simulink model "SWC_HALIN_CDD_type"  (R2021b)
settings: Solver=FixedStepDiscrete  StartTime=0.0  StopTime=10.0  FixedStep=0.005  RelTol=1e-3
undefined symbols (not defined in the file or in its folder): C_TASK_5MS_S, DIDLen_APSFunConfig, DIDLen_AutoLock, DIDLen_AutoWipHSpdEN, DIDLen_DKCKey, DIDLen_DRLDis, DIDLen_DynoMode, DIDLen_FMHTimer, DIDLen_OBDReq, DIDLen_TestGroup, DIDLen_TireSize, DIDLen_TurnLampFLThreCurr, DIDLen_TurnLampFRThreCurr, DIDLen_TurnLampRLThreCurr, DIDLen_TurnLampRRThreCurr, DIDLen_USSConfig, DIDLen_WipRLSCmdCutFilter, DIDLen_WipRLSCmdHoldFilter, DIDLen_XWDMode, DIDNum_APSFunConfig, DIDNum_AutoLock, DIDNum_AutoWipHSpdEN, DIDNum_DKCKey, DIDNum_DRLDis, DIDNum_DynoMode, DIDNum_FMHTimer, DIDNum_OBDReq, DIDNum_TestGroup, DIDNum_TireSize, DIDNum_TurnLampFLThreCurr, DIDNum_TurnLampFRThreCurr, DIDNum_TurnLampRLThreCurr, DIDNum_TurnLampRRThreCurr, DIDNum_USSConfig, DIDNum_WipRLSCmdCutFilter, DIDNum_WipRLSCmdHoldFilter, DIDNum_XWDMode, ENUM_DRIVETRAIN_AWD, ENUM_DRIVETRAIN_FWD, ENUM_DRIVETRAIN_RWD, ENUM_REGENLEVEL_LV1, ENUM_REGENLEVEL_LV2, ENUM_REGENLEVEL_LV3, ENUM_REGENLEVEL_LV4, ENUM_REGENLEVEL_LV5, ENUM_REGENLEVEL_OPD, ENUM_TPMSSTA_FAT, ENUM_TPMSSTA_LOWBATTERY, ENUM_TPMSSTA_TRIGGER, FALSE, FIVE_INT, FOUR_INT, KHAL_CANBusOffDebounce_s, KHAL_DefaultRegenMode_enum, KHAL_DKCDecryptEnable_flg_ovrdflg, KHAL_DKCDecryptEnable_flg_ovrdval, KHAL_RandomNumberY1_enum, KHAL_RandomNumberY2_enum, KHAL_RandomNumberY_ovrdflg, KHAL_TPMSRESBUTT_flg_ovrdflg ... (+9)
libraries: simulink x229, FVT_lib x29, hcu_lib x25, hdlsllib x15
(part 6 of 8)

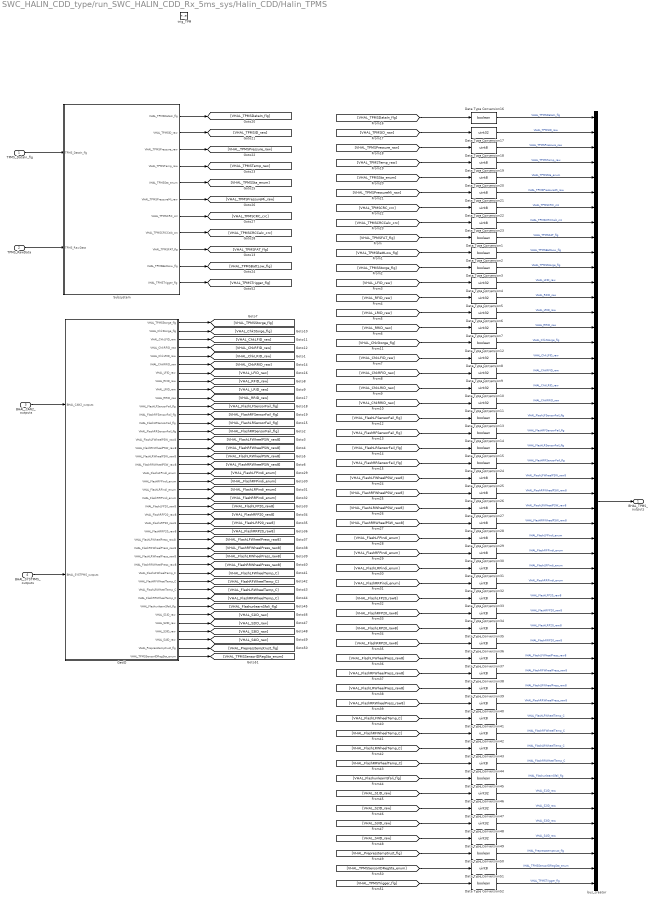
== system SWC_HALIN_CDD_type/run_SWC_HALIN_CDD_Rx_5ms_sys/Halin_CDD/Halin_TPMS ==
  TPMS_DataIn_flg : Inport
  TPMS_RawData : Inport  Port=2
  BHAL_CAN2_outputs : Inport  Port=3
  BHAL_SYSTPMS_outputs : Inport  Port=4
  trig_TPM : TriggerPort  TriggerType=function-call  VariantControl=(inherit)
  Data Type Conversion{1..3,12..16,24,45,50,52} (12 alike) : DataTypeConversion  OutDataTypeStr=boolean
  Data Type Conversion{4..11,17,46..49} (13 alike) : DataTypeConversion  OutDataTypeStr=uint32
  Data Type Conversion{18..23,25..44,51} (27 alike) : DataTypeConversion  OutDataTypeStr=uint8
  GetID : Subsystem
  Subsystem : Subsystem
  bus_creator : BusCreator  Inputs=52  OutDataTypeStr=Bus: BHAL_TPMS_outputs  NonVirtualBus=on
  BHAL_TPMS_outputs : Outport
  wires:
  TPMS_DataIn_flg/1 -> Subsystem/1(TPMS_DataIn_flg)
  Data Type Conversion29/1 -> bus_creator/29  "VHAL_FlashLFPindi_enum"
  GetID/20(VHAL_FlashRFPindi_enum) -> [VHAL_FlashRFPindi_enum]
  GetID/32(VHAL_FlashRFWheelTemp_C) -> [VHAL_FlashRFWheelTemp_C]
  Data Type Conversion2/1 -> bus_creator/10  "VHAL_TPMSBattLow_flg"
  BHAL_CAN2_outputs/1 -> GetID/1(BHAL_CAN2_outputs)
  [VHAL_TPMSBattLow_flg] -> Data Type Conversion2/1
  [VHAL_FlashLRPindi_enum] -> Data Type Conversion31/1
  [VHAL_FlashunlearnSfali_flg] -> Data Type Conversion45/1
  [VHAL_FlashLFPindi_enum] -> Data Type Conversion29/1
  Data Type Conversion28/1 -> bus_creator/28  "VHAL_FlashRRWheelPSW_raw8"
  [VHAL_FlashLFP20_raw8] -> Data Type Conversion33/1
  [VHAL_RRID_raw] -> Data Type Conversion7/1
  Data Type Conversion42/1 -> bus_creator/42  "VHAL_FlashRFWheelTemp_C"
  Data Type Conversion27/1 -> bus_creator/27  "VHAL_FlashLRWheelPSW_raw8"
  [VHAL_FlashLFWheelTemp_C] -> Data Type Conversion41/1
  Data Type Conversion26/1 -> bus_creator/26  "VHAL_FlashRFWheelPSW_raw8"
  [VHAL_FlashRRP20_raw8] -> Data Type Conversion36/1
  GetID/16(VHAL_FlashRFWheelPSW_raw8) -> [VHAL_FlashRFWheelPSW_raw8]
  [VHAL_RFID_raw] -> Data Type Conversion5/1
  Data Type Conversion33/1 -> bus_creator/33  "VHAL_FlashLFP20_raw8"
  Data Type Conversion24/1 -> bus_creator/24  "VHAL_FlashRRSensorFail_flg"
  Data Type Conversion44/1 -> bus_creator/44  "VHAL_FlashRRWheelTemp_C"
  Data Type Conversion34/1 -> bus_creator/34  "VHAL_FlashRFP20_raw8"
  Data Type Conversion45/1 -> bus_creator/45  "VHAL_FlashunlearnSfali_flg"
  GetID/9(VHAL_LRID_raw) -> [VHAL_LRID_raw]
  Data Type Conversion41/1 -> bus_creator/41  "VHAL_FlashLFWheelTemp_C"
  GetID/15(VHAL_FlashLFWheelPSW_raw8) -> [VHAL_FlashLFWheelPSW_raw8]
  Data Type Conversion15/1 -> bus_creator/23  "VHAL_FlashLRSensorFail_flg"
  [VHAL_FlashLRWheelPress_raw8] -> Data Type Conversion39/1
  Data Type Conversion14/1 -> bus_creator/22  "VHAL_FlashRFSensorFail_flg"
  GetID/34(VHAL_FlashRRWheelTemp_C) -> [VHAL_FlashRRWheelTemp_C]
  Data Type Conversion13/1 -> bus_creator/21  "VHAL_FlashLFSensorFail_flg"
  Data Type Conversion32/1 -> bus_creator/32  "VHAL_FlashRRPindi_enum"
  Data Type Conversion31/1 -> bus_creator/31  "VHAL_FlashLRPindi_enum"
  Data Type Conversion16/1 -> bus_creator/1  "VHAL_TPMSDataIn_flg"
  GetID/22(VHAL_FlashRRPindi_enum) -> [VHAL_FlashRRPindi_enum]
  [VHAL_FlashRFSensorFail_flg] -> Data Type Conversion14/1
  GetID/18(VHAL_FlashRRWheelPSW_raw8) -> [VHAL_FlashRRWheelPSW_raw8]
  Data Type Conversion43/1 -> bus_creator/43  "VHAL_FlashLRWheelTemp_C"
  Data Type Conversion22/1 -> bus_creator/7  "VHAL_TPMSCRC_crc"
  Data Type Conversion40/1 -> bus_creator/40  "VHAL_FlashRRWheelPress_raw8"
  Data Type Conversion39/1 -> bus_creator/39  "VHAL_FlashLRWheelPress_raw8"
  [VHAL_FlashRRPindi_enum] -> Data Type Conversion32/1
  Data Type Conversion38/1 -> bus_creator/38  "VHAL_FlashRFWheelPress_raw8"
  [VHAL_FlashLRP20_raw8] -> Data Type Conversion35/1
  Data Type Conversion35/1 -> bus_creator/35  "VHAL_FlashLRP20_raw8"
  GetID/14(VHAL_FlashRRSensorFail_flg) -> [VHAL_FlashRRSensorFail_flg]
  Data Type Conversion37/1 -> bus_creator/37  "VHAL_FlashLFWheelPress_raw8"
  Data Type Conversion36/1 -> bus_creator/36  "VHAL_FlashRRP20_raw8"
  [VHAL_FlashRRWheelTemp_C] -> Data Type Conversion44/1
  [VHAL_FlashLFWheelPress_raw8] -> Data Type Conversion37/1
  GetID/33(VHAL_FlashLRWheelTemp_C) -> [VHAL_FlashLRWheelTemp_C]
  GetID/26(VHAL_FlashRRP20_raw8) -> [VHAL_FlashRRP20_raw8]
  [VHAL_TPMSFAT_flg] -> Data Type Conversion1/1
  [VHAL_TPMSSta_enum] -> Data Type Conversion20/1
  GetID/25(VHAL_FlashLRP20_raw8) -> [VHAL_FlashLRP20_raw8]
  [VHAL_FlashRRWheelPress_raw8] -> Data Type Conversion40/1
  [VHAL_FlashRFP20_raw8] -> Data Type Conversion34/1
  [VHAL_LFID_raw] -> Data Type Conversion4/1
  [VHAL_FlashRFWheelPSW_raw8] -> Data Type Conversion26/1
  [VHAL_FlashRFWheelTemp_C] -> Data Type Conversion42/1
  [VHAL_FlashLRWheelTemp_C] -> Data Type Conversion43/1
  [VHAL_TPMSCRCCalc_crc] -> Data Type Conversion23/1
  GetID/31(VHAL_FlashLFWheelTemp_C) -> [VHAL_FlashLFWheelTemp_C]
  [VHAL_FlashRRSensorFail_flg] -> Data Type Conversion24/1
  [VHAL_FlashLFSensorFail_flg] -> Data Type Conversion13/1
  GetID/30(VHAL_FlashRRWheelPress_raw8) -> [VHAL_FlashRRWheelPress_raw8]
  Data Type Conversion3/1 -> bus_creator/11  "VHAL_TPMSStorge_flg"
  GetID/29(VHAL_FlashLRWheelPress_raw8) -> [VHAL_FlashLRWheelPress_raw8]
  GetID/21(VHAL_FlashLRPindi_enum) -> [VHAL_FlashLRPindi_enum]
  GetID/1(VHAL_TPMSStorge_flg) -> [VHAL_TPMSStorge_flg]
  [VHAL_FlashRFPindi_enum] -> Data Type Conversion30/1
  GetID/19(VHAL_FlashLFPindi_enum) -> [VHAL_FlashLFPindi_enum]
  GetID/23(VHAL_FlashLFP20_raw8) -> [VHAL_FlashLFP20_raw8]
  Data Type Conversion6/1 -> bus_creator/14  "VHAL_LRID_raw"
  GetID/6(VHAL_ChkRRID_raw) -> [VHAL_ChkRRID_raw]
  [VHAL_TPMSDataIn_flg] -> Data Type Conversion16/1
  GetID/17(VHAL_FlashLRWheelPSW_raw8) -> [VHAL_FlashLRWheelPSW_raw8]
  [VHAL_FlashRFWheelPress_raw8] -> Data Type Conversion38/1
  Data Type Conversion1/1 -> bus_creator/9  "VHAL_TPMSFAT_flg"
  GetID/3(VHAL_ChkLFID_raw) -> [VHAL_ChkLFID_raw]
  GetID/35(VHAL_FlashunlearnSfali_flg) -> [VHAL_FlashunlearnSfali_flg]
  [VHAL_FlashLFWheelPSW_raw8] -> Data Type Conversion25/1
  GetID/8(VHAL_RFID_raw) -> [VHAL_RFID_raw]
  GetID/10(VHAL_RRID_raw) -> [VHAL_RRID_raw]
  Data Type Conversion12/1 -> bus_creator/16  "VHAL_ChkStorge_flg"
  [VHAL_FlashLRWheelPSW_raw8] -> Data Type Conversion27/1
  GetID/7(VHAL_LFID_raw) -> [VHAL_LFID_raw]
  Data Type Conversion18/1 -> bus_creator/3  "VHAL_TPMSPressure_raw"
  Data Type Conversion9/1 -> bus_creator/18  "VHAL_ChkRFID_raw"
  Data Type Conversion10/1 -> bus_creator/19  "VHAL_ChkLRID_raw"
  GetID/11(VHAL_FlashLFSensorFail_flg) -> [VHAL_FlashLFSensorFail_flg]
  GetID/27(VHAL_FlashLFWheelPress_raw8) -> [VHAL_FlashLFWheelPress_raw8]
  Data Type Conversion11/1 -> bus_creator/20  "VHAL_ChkRRID_raw"
  Data Type Conversion7/1 -> bus_creator/15  "VHAL_RRID_raw"
  GetID/4(VHAL_ChkRFID_raw) -> [VHAL_ChkRFID_raw]
  [VHAL_TPMSID_raw] -> Data Type Conversion17/1
  [VHAL_ChkStorge_flg] -> Data Type Conversion12/1
  GetID/28(VHAL_FlashRFWheelPress_raw8) -> [VHAL_FlashRFWheelPress_raw8]
  Data Type Conversion8/1 -> bus_creator/17  "VHAL_ChkLFID_raw"
  [VHAL_ChkRRID_raw] -> Data Type Conversion11/1
  Data Type Conversion4/1 -> bus_creator/12  "VHAL_LFID_raw"
  [VHAL_ChkLRID_raw] -> Data Type Conversion10/1
  [VHAL_ChkLFID_raw] -> Data Type Conversion8/1
  [VHAL_ChkRFID_raw] -> Data Type Conversion9/1
  Data Type Conversion5/1 -> bus_creator/13  "VHAL_RFID_raw"
  [VHAL_LRID_raw] -> Data Type Conversion6/1
  [VHAL_TPMSStorge_flg] -> Data Type Conversion3/1
  GetID/2(VHAL_ChkStorge_flg) -> [VHAL_ChkStorge_flg]
  [VHAL_TPMSCRC_crc] -> Data Type Conversion22/1
  Data Type Conversion19/1 -> bus_creator/4  "VHAL_TPMSTemp_raw"
  BHAL_SYSTPMS_outputs/1 -> GetID/2(BHAL_SYSTPMS_outputs)
  [VHAL_FlashLRSensorFail_flg] -> Data Type Conversion15/1
  Data Type Conversion17/1 -> bus_creator/2  "VHAL_TPMSID_raw"
  Data Type Conversion23/1 -> bus_creator/8  "VHAL_TPMSCRCCalc_crc"
  Data Type Conversion30/1 -> bus_creator/30  "VHAL_FlashRFPindi_enum"
  Data Type Conversion21/1 -> bus_creator/6  "VHAL_TPMSPressureMi_raw"
  GetID/5(VHAL_ChkLRID_raw) -> [VHAL_ChkLRID_raw]
  [VHAL_TPMSTemp_raw] -> Data Type Conversion19/1
  GetID/13(VHAL_FlashLRSensorFail_flg) -> [VHAL_FlashLRSensorFail_flg]
  [VHAL_TPMSPressure_raw] -> Data Type Conversion18/1
  GetID/24(VHAL_FlashRFP20_raw8) -> [VHAL_FlashRFP20_raw8]
  bus_creator/1 -> BHAL_TPMS_outputs/1
  Data Type Conversion20/1 -> bus_creator/5  "VHAL_TPMSSta_enum"
  Data Type Conversion25/1 -> bus_creator/25  "VHAL_FlashLFWheelPSW_raw8"
  [VHAL_TPMSPressureMi_raw] -> Data Type Conversion21/1
  GetID/12(VHAL_FlashRFSensorFail_flg) -> [VHAL_FlashRFSensorFail_flg]
  [VHAL_FlashRRWheelPSW_raw8] -> Data Type Conversion28/1
  GetID/36(VHAL_S1ID_raw) -> [VHAL_S1ID_raw]
  GetID/37(VHAL_S2ID_raw) -> [VHAL_S2ID_raw]
  GetID/38(VHAL_S3ID_raw) -> [VHAL_S3ID_raw]
  GetID/39(VHAL_S4ID_raw) -> [VHAL_S4ID_raw]
  Data Type Conversion46/1 -> bus_creator/46  "VHAL_S1ID_raw"
  Data Type Conversion49/1 -> bus_creator/49  "VHAL_S4ID_raw"
  Data Type Conversion48/1 -> bus_creator/48  "VHAL_S3ID_raw"
  Data Type Conversion47/1 -> bus_creator/47  "VHAL_S2ID_raw"
  [VHAL_S1ID_raw] -> Data Type Conversion46/1
  [VHAL_S2ID_raw] -> Data Type Conversion47/1
  [VHAL_S3ID_raw] -> Data Type Conversion48/1
  [VHAL_S4ID_raw] -> Data Type Conversion49/1
  GetID/40(VHAL_Prepresstemptrust_flg) -> [VHAL_Prepresstemptrust_flg]
  [VHAL_Prepresstemptrust_flg] -> Data Type Conversion50/1
  Data Type Conversion50/1 -> bus_creator/50  "VHAL_Prepresstemptrust_flg"
  GetID/41(VHAL_TPMSSensorIDRegSta_enum) -> [VHAL_TPMSSensorIDRegSta_enum]
  [VHAL_TPMSSensorIDRegSta_enum] -> Data Type Conversion51/1
  Data Type Conversion51/1 -> bus_creator/51  "VHAL_TPMSSensorIDRegSta_enum"
  Subsystem/11(VHAL_TPMSTrigger_flg) -> [VHAL_TPMSTrigger_flg]
  Data Type Conversion52/1 -> bus_creator/52  "VHAL_TPMSTrigger_flg"
  [VHAL_TPMSTrigger_flg] -> Data Type Conversion52/1
  TPMS_RawData/1 -> Subsystem/2(TPMS_RawData)
  Subsystem/1(VHAL_TPMSDataIn_flg) -> [VHAL_TPMSDataIn_flg]
  Subsystem/2(VHAL_TPMSID_raw) -> [VHAL_TPMSID_raw]
  Subsystem/3(VHAL_TPMSPressure_raw) -> [VHAL_TPMSPressure_raw]
  Subsystem/4(VHAL_TPMSTemp_raw) -> [VHAL_TPMSTemp_raw]
  Subsystem/5(VHAL_TPMSSta_enum) -> [VHAL_TPMSSta_enum]
  Subsystem/6(VHAL_TPMSPressureMi_raw) -> [VHAL_TPMSPressureMi_raw]
  Subsystem/7(VHAL_TPMSCRC_crc) -> [VHAL_TPMSCRC_crc]
  Subsystem/8(VHAL_TPMSCRCCalc_crc) -> [VHAL_TPMSCRCCalc_crc]
  Subsystem/9(VHAL_TPMSFAT_flg) -> [VHAL_TPMSFAT_flg]
  Subsystem/10(VHAL_TPMSBattLow_flg) -> [VHAL_TPMSBattLow_flg]

== system SWC_HALIN_CDD_type/run_SWC_HALIN_CDD_Rx_5ms_sys/Halin_CDD/Subsystem ==
  VHAL_ClearDTCcmd_flg : Inport
  VHAL_ClearZevDTCcmd_flg : Inport  Port=2
  Bus Creator : BusCreator  Inputs=2  OutDataTypeStr=Bus: BHAL_DDM_outputs  NonVirtualBus=on
  Data Type Conversion : DataTypeConversion  OutDataTypeStr=boolean
  Data Type Conversion1 : DataTypeConversion  OutDataTypeStr=boolean
  BHAL_DDM_outputs : Outport  OutDataTypeStr=Bus: BHAL_DDM_outputs
  wires:
  VHAL_ClearDTCcmd_flg/1 -> Data Type Conversion/1
  Bus Creator/1 -> BHAL_DDM_outputs/1
  Data Type Conversion/1 -> Bus Creator/1  "VHAL_ClearDTCcmd_flg"
  Data Type Conversion1/1 -> Bus Creator/2  "VHAL_ClearZevDTCcmd_flg"
  VHAL_ClearZevDTCcmd_flg/1 -> Data Type Conversion1/1

== system SWC_HALIN_CDD_type/run_SWC_HALIN_CDD_Rx_5ms_sys/Halin_CDD/Subsystem7 ==
  u8Array17_VinCode : Inport
  Data Type Conversion{,1..16} (17 alike) : DataTypeConversion
  Demux : Demux  Outputs=17
  Display{1..17} (17 alike) : Display
  wires:
  Demux/1 -> Data Type Conversion/1
  u8Array17_VinCode/1 -> Demux/1
  Data Type Conversion/1 -> Display1/1  "VINP_VinCodeByte0_enum"
  Data Type Conversion1/1 -> Display2/1  "VINP_VinCodeByte1_enum"
  Demux/2 -> Data Type Conversion1/1
  Demux/3 -> Data Type Conversion2/1
  Demux/4 -> Data Type Conversion3/1
  Demux/5 -> Data Type Conversion4/1
  Demux/6 -> Data Type Conversion5/1
  Demux/7 -> Data Type Conversion6/1
  Data Type Conversion2/1 -> Display3/1  "VINP_VinCodeByte2_enum"
  Data Type Conversion3/1 -> Display4/1  "VINP_VinCodeByte3_enum"
  Data Type Conversion4/1 -> Display5/1  "VINP_VinCodeByte4_enum"
  Data Type Conversion5/1 -> Display6/1  "VINP_VinCodeByte5_enum"
  Data Type Conversion6/1 -> Display7/1  "VINP_VinCodeByte6_enum"
  Demux/8 -> Data Type Conversion7/1
  Demux/9 -> Data Type Conversion8/1
  Demux/10 -> Data Type Conversion9/1
  Demux/11 -> Data Type Conversion10/1
  Demux/12 -> Data Type Conversion11/1
  Demux/13 -> Data Type Conversion12/1
  Demux/14 -> Data Type Conversion13/1
  Demux/15 -> Data Type Conversion14/1
  Demux/16 -> Data Type Conversion15/1
  Demux/17 -> Data Type Conversion16/1
  Data Type Conversion7/1 -> Display8/1  "VINP_VinCodeByte7_enum"
  Data Type Conversion8/1 -> Display9/1  "VINP_VinCodeByte8_enum"
  Data Type Conversion9/1 -> Display10/1  "VINP_VinCodeByte9_enum"
  Data Type Conversion10/1 -> Display11/1  "VINP_VinCodeByte10_enum"
  Data Type Conversion11/1 -> Display12/1  "VINP_VinCodeByte11_enum"
  Data Type Conversion12/1 -> Display13/1  "VINP_VinCodeByte12_enum"
  Data Type Conversion13/1 -> Display14/1  "VINP_VinCodeByte13_enum"
  Data Type Conversion14/1 -> Display15/1  "VINP_VinCodeByte14_enum"
  Data Type Conversion15/1 -> Display16/1  "VINP_VinCodeByte15_enum"
  Data Type Conversion16/1 -> Display17/1  "VINP_VinCodeByte16_enum"

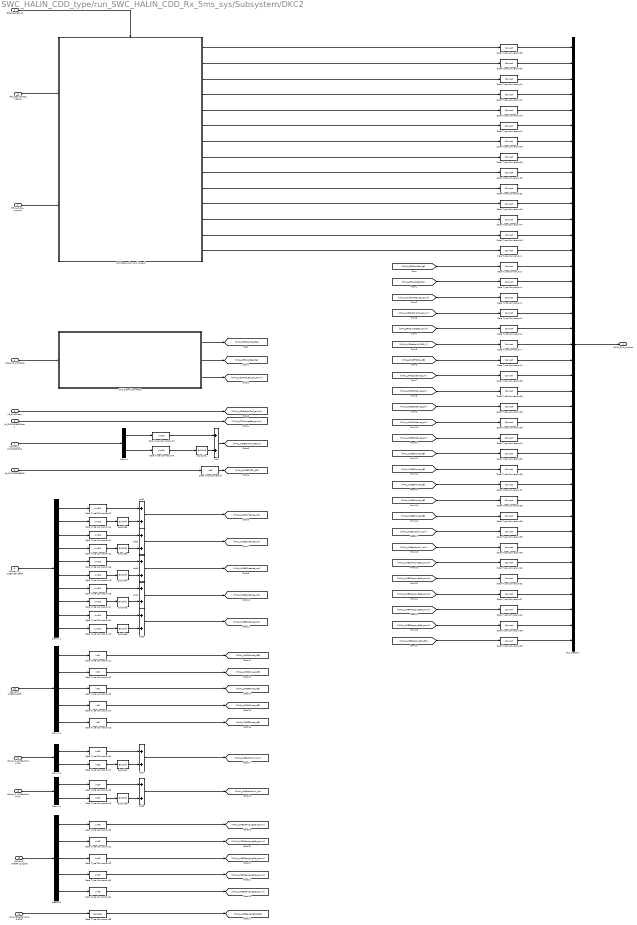
== system SWC_HALIN_CDD_type/run_SWC_HALIN_CDD_Rx_5ms_sys/Subsystem/DKC2 ==
  Enable_Decrypt : Inport
  DKC_ResultData_16byte : Inport  Port=2
  BHAL_CAN4_outputs : Inport  Port=3
  u8Array3_DKCData : Inport  Port=4
  u8_DKCButton : Inport  Port=5
  u8_DKCUIDBLEStatus : Inport  Port=6
  u8Array2_DKCUIDBLEVol : Inport  Port=7
  s8_DKCUIDBLERSSI : Inport  Port=8
  u8Array10_UWBDistanceCM : Inport  Port=9
  s8Array5_UWBPowerdB : Inport  Port=10
  s8Array2_UWBpositionXCM : Inport  Port=11
  s8Array2_UWBpositionYCM : Inport  Port=12
  u8Array5_UWBRangingSta : Inport  Port=13
  u8_UWBStaRangingONOFF : Inport  Port=14
  Add{,1..7} (8 alike) : Sum
  Bit Shift{1..8} (8 alike) : hdlsllib/Logic and Bit Operations/Bit Shift  mode=Shift Left Logical  N=8
  Bus Creator1 : BusCreator  Inputs=39  OutDataTypeStr=Bus: BHAL_DKC_outputs  NonVirtualBus=on
  DKC Decryption and Unpack : Subsystem
  DKC Signal Convertor : Subsystem
  Data Type Conversion{,21..25} (6 alike) : DataTypeConversion  OutDataTypeStr=int8
  Data Type Conversion{1..8,35..65} (39 alike) : DataTypeConversion
  Data Type Conversion{9..20} (12 alike) : DataTypeConversion  OutDataTypeStr=uint16
  Data Type Conversion{26..29} (4 alike) : DataTypeConversion  OutDataTypeStr=int16
  Data Type Conversion{30..34} (5 alike) : DataTypeConversion  OutDataTypeStr=uint8
  Data Type Conversion66 : DataTypeConversion  OutDataTypeStr=boolean
  Demux : Demux  Outputs=2
  Demux1 : Demux  Outputs=10
  Demux2 : Demux  Outputs=5
  Demux3 : Demux  Outputs=2
  Demux4 : Demux  Outputs=2
  Demux5 : Demux  Outputs=5
  BHAL_DKC_outputs : Outport
  wires:
  DKC Decryption and Unpack/1(VHAL_DKCDecReVehData_enum) -> Data Type Conversion53/1
  DKC Decryption and Unpack/2(VHAL_DKCDecRemotePW_enum) -> Data Type Conversion54/1
  DKC Decryption and Unpack/3(VHAL_DKCDecPCommandToBCM_enum) -> Data Type Conversion41/1
  DKC Decryption and Unpack/4(VHAL_DKCDecPCommandToPTG_enum) -> Data Type Conversion42/1
  DKC Decryption and Unpack/5(VHAL_DKCDecPDKeyAreaLockUnlock_enum) -> Data Type Conversion43/1
  DKC Decryption and Unpack/6(VHAL_DKCDecPDKeyAreaPS_enum) -> Data Type Conversion44/1
  DKC Decryption and Unpack/7(VHAL_DKCDecPDKeyAreaPTG_enum) -> Data Type Conversion45/1
  DKC Decryption and Unpack/8(VHAL_DKCDecPDKeyWelcome_enum) -> Data Type Conversion49/1
  DKC Decryption and Unpack/13(VHAL_TimeSNDKCFbk_cnt) -> Data Type Conversion48/1
  DKC Decryption and Unpack/9(VHAL_DKCDecPDkeyShowIVI_enum) -> Data Type Conversion50/1
  DKC Decryption and Unpack/12(VHAL_DKCDecPUIDLowPower_flg) -> Data Type Conversion47/1
  DKC Decryption and Unpack/10(VHAL_DKCDecPKeyMiss_flg) -> Data Type Conversion51/1
  DKC Decryption and Unpack/11(VHAL_DKCDecPKeyMode_enum) -> Data Type Conversion46/1
  Data Type Conversion43/1 -> Bus Creator1/5  "VHAL_DKCDecPDKeyAreaLockUnlock_enum"
  Data Type Conversion54/1 -> Bus Creator1/2  "VHAL_DKCDecRemotePW_enum"
  Data Type Conversion53/1 -> Bus Creator1/1  "VHAL_DKCDecReVehData_enum"
  Data Type Conversion41/1 -> Bus Creator1/3  "VHAL_DKCDecPCommandToBCM_enum"
  Data Type Conversion46/1 -> Bus Creator1/11  "VHAL_DKCDecPKeyMode_enum"
  Data Type Conversion47/1 -> Bus Creator1/12  "VHAL_DKCDecPUIDLowPower_flg"
  Data Type Conversion42/1 -> Bus Creator1/4  "VHAL_DKCDecPCommandToPTG_enum"
  Data Type Conversion50/1 -> Bus Creator1/9  "VHAL_DKCDecPDkeyShowIVI_enum"
  Bus Creator1/1 -> BHAL_DKC_outputs/1  "BHAL_DKC_outputs"
  Data Type Conversion51/1 -> Bus Creator1/10  "VHAL_DKCDecPKeyMiss_flg"
  Data Type Conversion49/1 -> Bus Creator1/8  "VHAL_DKCDecPDKeyWelcome_enum"
  Data Type Conversion48/1 -> Bus Creator1/13  "VHAL_TimeSNDKCFbk_cnt"
  Data Type Conversion45/1 -> Bus Creator1/7  "VHAL_DKCDecPDKeyAreaPTG_enum"
  Data Type Conversion44/1 -> Bus Creator1/6  "VHAL_DKCDecPDKeyAreaPS_enum"
  Enable_Decrypt/1 -> DKC Decryption and Unpack/Enable
  DKC_ResultData_16byte/1 -> DKC Decryption and Unpack/1(DKC_ResultData_16byte)
  DKC Decryption and Unpack/14(VHAL_DKCDecryptionFail_flg) -> Data Type Conversion1/1
  Data Type Conversion1/1 -> Bus Creator1/14  "VHAL_DKCDecryptionFail_flg"
  BHAL_CAN4_outputs/1 -> DKC Decryption and Unpack/2(BHAL_CAN4_outputs)
  u8Array3_DKCData/1 -> DKC Signal Convertor/1(u8Array3_DKCData)
  Data Type Conversion3/1 -> Bus Creator1/15  "VHAL_NFCDoorSta_flg"
  Data Type Conversion4/1 -> Bus Creator1/16  "VHAL_NFCLidASta_flg"
  Data Type Conversion2/1 -> Bus Creator1/17  "VHAL_KeyFobAreaU16_enum"
  DKC Signal Convertor/2(VHAL_NFCLidASta_flg) -> [VHAL_NFCLidASta_flg]
  DKC Signal Convertor/1(VHAL_NFCDoorSta_flg) -> [VHAL_NFCDoorSta_flg]
  DKC Signal Convertor/3(VHAL_KeyFobAreaU16_enum) -> [VHAL_KeyFobAreaU16_enum]
  [VHAL_NFCDoorSta_flg] -> Data Type Conversion3/1
  [VHAL_NFCLidASta_flg] -> Data Type Conversion4/1
  [VHAL_KeyFobAreaU16_enum] -> Data Type Conversion2/1
  Data Type Conversion5/1 -> Bus Creator1/18  "VHAL_UIDButtonCmd_enum"
  [VHAL_UIDButtonCmd_enum] -> Data Type Conversion5/1
  u8_DKCButton/1 -> [VHAL_UIDButtonCmd_enum]
  s8_DKCUIDBLERSSI/1 -> Data Type Conversion/1
  Data Type Conversion10/1 -> Add/1
  u8_DKCUIDBLEStatus/1 -> [VHAL_BTConnectSta_enum]
  Data Type Conversion/1 -> [VHAL_DKCBTRSSI_dB]
  Add/1 -> [VHAL_UIDBatVoltx1000_V]
  Bit Shift1/1 -> Add/2
  u8Array2_DKCUIDBLEVol/1 -> Demux/1
  Demux/1 -> Data Type Conversion10/1
  Demux/2 -> Data Type Conversion9/1
  Data Type Conversion9/1 -> Bit Shift1/1
  [VHAL_BTConnectSta_enum] -> Data Type Conversion6/1
  Data Type Conversion6/1 -> Bus Creator1/19  "VHAL_BTConnectSta_enum"
  Data Type Conversion7/1 -> Bus Creator1/20  "VHAL_UIDBatVoltx1000_V"
  Data Type Conversion8/1 -> Bus Creator1/21  "VHAL_DKCBTRSSI_dB"
  [VHAL_UIDBatVoltx1000_V] -> Data Type Conversion7/1
  [VHAL_DKCBTRSSI_dB] -> Data Type Conversion8/1
  u8Array10_UWBDistanceCM/1 -> Demux1/1
  Add1/1 -> [VHAL_UWB1Distance_cm]
  Data Type Conversion11/1 -> Bit Shift2/1
  Bit Shift2/1 -> Add1/2
  Data Type Conversion12/1 -> Add1/1
  Demux1/1 -> Data Type Conversion12/1
  Demux1/2 -> Data Type Conversion11/1
  Demux1/4 -> Data Type Conversion13/1
  Demux1/3 -> Data Type Conversion14/1
  Data Type Conversion14/1 -> Add2/1
  Bit Shift3/1 -> Add2/2
  Data Type Conversion13/1 -> Bit Shift3/1
  Add2/1 -> [VHAL_UWB2Distance_cm]
  Add3/1 -> [VHAL_UWB3Distance_cm]
  Data Type Conversion15/1 -> Bit Shift4/1
  Bit Shift4/1 -> Add3/2
  Data Type Conversion16/1 -> Add3/1
  Demux1/5 -> Data Type Conversion16/1
  Demux1/6 -> Data Type Conversion15/1
  Demux1/8 -> Data Type Conversion17/1
  Demux1/7 -> Data Type Conversion18/1
  Data Type Conversion18/1 -> Add4/1
  Bit Shift5/1 -> Add4/2
  Data Type Conversion17/1 -> Bit Shift5/1
  Add4/1 -> [VHAL_UWB4Distance_cm]
  Add5/1 -> [VHAL_UWB5Distance_cm]
  Data Type Conversion19/1 -> Bit Shift6/1
  Bit Shift6/1 -> Add5/2
  Data Type Conversion20/1 -> Add5/1
  Demux1/9 -> Data Type Conversion20/1
  Demux1/10 -> Data Type Conversion19/1
  s8Array5_UWBPowerdB/1 -> Demux2/1
  Demux2/1 -> Data Type Conversion21/1
  Demux2/2 -> Data Type Conversion22/1
  Demux2/3 -> Data Type Conversion23/1
  Demux2/4 -> Data Type Conversion24/1
  Demux2/5 -> Data Type Conversion25/1
  Data Type Conversion21/1 -> [VHAL_UWB1Power_dB]
  Data Type Conversion22/1 -> [VHAL_UWB2Power_dB]
  Data Type Conversion23/1 -> [VHAL_UWB3Power_dB]
  Data Type Conversion24/1 -> [VHAL_UWB4Power_dB]
  Data Type Conversion25/1 -> [VHAL_UWB5Power_dB]
  s8Array2_UWBpositionXCM/1 -> Demux3/1
  Demux3/1 -> Data Type Conversion26/1
  Demux3/2 -> Data Type Conversion27/1
  Data Type Conversion27/1 -> Bit Shift7/1
  Bit Shift7/1 -> Add7/2
  Data Type Conversion26/1 -> Add7/1
  Add7/1 -> [VHAL_UWBpositionX_cm]
  Add6/1 -> [VHAL_UWBpositionY_cm]
  Data Type Conversion28/1 -> Add6/1
  Bit Shift8/1 -> Add6/2
  Data Type Conversion29/1 -> Bit Shift8/1
  Demux4/2 -> Data Type Conversion29/1
  Demux4/1 -> Data Type Conversion28/1
  s8Array2_UWBpositionYCM/1 -> Demux4/1
  Data Type Conversion34/1 -> [VHAL_UWB5RangingSta_enum]
  Data Type Conversion33/1 -> [VHAL_UWB4RangingSta_enum]
  Data Type Conversion32/1 -> [VHAL_UWB3RangingSta_enum]
  Data Type Conversion31/1 -> [VHAL_UWB2RangingSta_enum]
  Data Type Conversion30/1 -> [VHAL_UWB1RangingSta_enum]
  Demux5/5 -> Data Type Conversion34/1
  Demux5/4 -> Data Type Conversion33/1
  Demux5/3 -> Data Type Conversion32/1
  Demux5/2 -> Data Type Conversion31/1
  Demux5/1 -> Data Type Conversion30/1
  u8Array5_UWBRangingSta/1 -> Demux5/1
  Data Type Conversion35/1 -> Bus Creator1/22  "VHAL_UWB1Distance_cm"
  [VHAL_UWB1Distance_cm] -> Data Type Conversion35/1
  Data Type Conversion64/1 -> Bus Creator1/37  "VHAL_UWB4RangingSta_enum"
  Data Type Conversion65/1 -> Bus Creator1/38  "VHAL_UWB5RangingSta_enum"
  Data Type Conversion63/1 -> Bus Creator1/39  "VHAL_UWBRangingON_flg"
  Data Type Conversion38/1 -> Bus Creator1/23  "VHAL_UWB2Distance_cm"
  Data Type Conversion36/1 -> Bus Creator1/24  "VHAL_UWB3Distance_cm"
  Data Type Conversion39/1 -> Bus Creator1/25  "VHAL_UWB4Distance_cm"
  Data Type Conversion40/1 -> Bus Creator1/26  "VHAL_UWB5Distance_cm"
  Data Type Conversion52/1 -> Bus Creator1/27  "VHAL_UWB1Power_dB"
  Data Type Conversion55/1 -> Bus Creator1/28  "VHAL_UWB2Power_dB"
  Data Type Conversion37/1 -> Bus Creator1/29  "VHAL_UWB3Power_dB"
  Data Type Conversion58/1 -> Bus Creator1/30  "VHAL_UWB4Power_dB"
  Data Type Conversion56/1 -> Bus Creator1/31  "VHAL_UWB5Power_dB"
  Data Type Conversion59/1 -> Bus Creator1/32  "VHAL_UWBpositionX_cm"
  Data Type Conversion60/1 -> Bus Creator1/33  "VHAL_UWBpositionY_cm"
  Data Type Conversion61/1 -> Bus Creator1/34  "VHAL_UWB1RangingSta_enum"
  Data Type Conversion62/1 -> Bus Creator1/35  "VHAL_UWB2RangingSta_enum"
  Data Type Conversion57/1 -> Bus Creator1/36  "VHAL_UWB3RangingSta_enum"
  [VHAL_UWB3Distance_cm] -> Data Type Conversion36/1
  [VHAL_UWB4Distance_cm] -> Data Type Conversion39/1
  [VHAL_UWB5Distance_cm] -> Data Type Conversion40/1
  [VHAL_UWB1Power_dB] -> Data Type Conversion52/1
  [VHAL_UWB2Power_dB] -> Data Type Conversion55/1
  [VHAL_UWB3Power_dB] -> Data Type Conversion37/1
  [VHAL_UWB4Power_dB] -> Data Type Conversion58/1
  [VHAL_UWB5Power_dB] -> Data Type Conversion56/1
  [VHAL_UWBpositionX_cm] -> Data Type Conversion59/1
  [VHAL_UWBpositionY_cm] -> Data Type Conversion60/1
  [VHAL_UWB1RangingSta_enum] -> Data Type Conversion61/1
  [VHAL_UWB2RangingSta_enum] -> Data Type Conversion62/1
  [VHAL_UWB3RangingSta_enum] -> Data Type Conversion57/1
  [VHAL_UWB4RangingSta_enum] -> Data Type Conversion64/1
  [VHAL_UWB5RangingSta_enum] -> Data Type Conversion65/1
  [VHAL_UWBRangingON_flg] -> Data Type Conversion63/1
  [VHAL_UWB2Distance_cm] -> Data Type Conversion38/1
  u8_UWBStaRangingONOFF/1 -> Data Type Conversion66/1
  Data Type Conversion66/1 -> [VHAL_UWBRangingON_flg]

== system SWC_HALIN_CDD_type/run_SWC_HALIN_CDD_Rx_5ms_sys/Halin_CDD/Halin_APM/Subsystem ==
  PASDistanceData : Inport
  APSDistanceData : Inport  Port=2
  APSLevelData : Inport  Port=3
  APSFaultStaData : Inport  Port=4
  ChimeIn : Inport  Port=5
  SNSRLayoutIn : Inport  Port=6
  StaFSyaIn : Inport  Port=7
  ModOperationIn : Inport  Port=8
  Demux : Demux  Outputs=8
  Demux1 : Demux  Outputs=12
  Demux2 : Demux  Outputs=8
  Demux3 : Demux
  PASDFCR : Outport
  PASDFMR : Outport  Port=2
  PASDFML : Outport  Port=3
  PASDFCL : Outport  Port=4
  PASDRCR : Outport  Port=5
  PASDRMR : Outport  Port=6
  PASDRML : Outport  Port=7
  PASDRCL : Outport  Port=8
  APSDFLL : Outport  Port=9
  APSDRLL : Outport  Port=10
  APSDFLR : Outport  Port=11
  APSDRLR : Outport  Port=12
  PASAFCR : Outport  Port=13
  PASAFMR : Outport  Port=14
  PASAFML : Outport  Port=15
  PASAFCL : Outport  Port=16
  PASARCR : Outport  Port=17
  PASARMR : Outport  Port=18
  PASARML : Outport  Port=19
  PASARCL : Outport  Port=20
  USSStaFCR : Outport  Port=21
  USSStaFMR : Outport  Port=22
  USSStaFML : Outport  Port=23
  USSStaFCL : Outport  Port=24
  USSStaRCR : Outport  Port=25
  USSStaRMR : Outport  Port=26
  USSStaRML : Outport  Port=27
  USSStaRCL : Outport  Port=28
  USSStaFLL : Outport  Port=29
  USSStaRLL : Outport  Port=30
  USSStaFLR : Outport  Port=31
  USSStaRLR : Outport  Port=32
  Chime : Outport  Port=33
  SNSRLayout : Outport  Port=34
  StaFSya : Outport  Port=35
  ModOperation : Outport  Port=36
  wires:
  Demux/8 -> [PASDRCL]
  Demux/7 -> [PASDRML]
  Demux/6 -> [PASDRMR]
  Demux/5 -> [PASDRCR]
  Demux/4 -> [PASDFCL]
  Demux/3 -> [PASDFML]
  Demux/2 -> [PASDFMR]
  Demux/1 -> [PASDFCR]
  [PASDRML] -> PASDRML/1
  [PASDRLR] -> APSDRLR/1
  [PASDFMR] -> PASDFMR/1
  [PASDFCL] -> PASDFCL/1
  [PASDRCL] -> PASDRCL/1
  [PASDRMR] -> PASDRMR/1
  [PASDRCR] -> PASDRCR/1
  [PASDFLL] -> APSDFLL/1
  [PASDFLR] -> APSDFLR/1
  [PASDRLL] -> APSDRLL/1
  [PASDFML] -> PASDFML/1
  Demux1/1 -> [USSStaFCR]
  ModOperationIn/1 -> ModOperation/1
  SNSRLayoutIn/1 -> SNSRLayout/1
  [PASDistanceData] -> Demux/1
  [PASDFCR] -> PASDFCR/1
  ChimeIn/1 -> Chime/1
  Demux1/2 -> [USSStaFMR]
  StaFSyaIn/1 -> StaFSya/1
  [APSFaultStaData] -> Demux1/1
  [APSLevelData] -> Demux2/1
  Demux2/1 -> [PASAFCR]
  Demux2/2 -> [PASAFMR]
  Demux2/3 -> [PASAFML]
  Demux2/4 -> [PASAFCL]
  Demux2/5 -> [PASARCR]
  Demux2/6 -> [PASARMR]
  Demux2/7 -> [PASARML]
  Demux2/8 -> [PASARCL]
  [PASAFCR] -> PASAFCR/1
  [PASAFMR] -> PASAFMR/1
  [PASAFML] -> PASAFML/1
  [PASAFCL] -> PASAFCL/1
  [PASARCR] -> PASARCR/1
  [PASARMR] -> PASARMR/1
  [PASARML] -> PASARML/1
  [PASARCL] -> PASARCL/1
  Demux1/3 -> [USSStaFML]
  Demux1/4 -> [USSStaFCL]
  Demux1/6 -> [USSStaRMR]
  Demux1/7 -> [USSStaRML]
  Demux1/9 -> [USSStaFLL]
  Demux1/10 -> [USSStaRLL]
  Demux1/12 -> [USSStaRLR]
  Demux1/11 -> [USSStaFLR]
  Demux1/5 -> [USSStaRCR]
  Demux1/8 -> [USSStaRCL]
  [USSStaFCR] -> USSStaFCR/1
  [USSStaFMR] -> USSStaFMR/1
  [USSStaFML] -> USSStaFML/1
  [USSStaFCL] -> USSStaFCL/1
  [USSStaRCR] -> USSStaRCR/1
  [USSStaRMR] -> USSStaRMR/1
  [USSStaRML] -> USSStaRML/1
  [USSStaRCL] -> USSStaRCL/1
  [USSStaFLL] -> USSStaFLL/1
  [USSStaRLL] -> USSStaRLL/1
  [USSStaFLR] -> USSStaFLR/1
  [USSStaRLR] -> USSStaRLR/1
  APSDistanceData/1 -> [APSDistanceData]
  APSLevelData/1 -> [APSLevelData]
  APSFaultStaData/1 -> [APSFaultStaData]
  PASDistanceData/1 -> [PASDistanceData]
  [APSDistanceData] -> Demux3/1
  Demux3/1 -> [PASDFLL]
  Demux3/2 -> [PASDRLL]
  Demux3/3 -> [PASDFLR]
  Demux3/4 -> [PASDRLR]

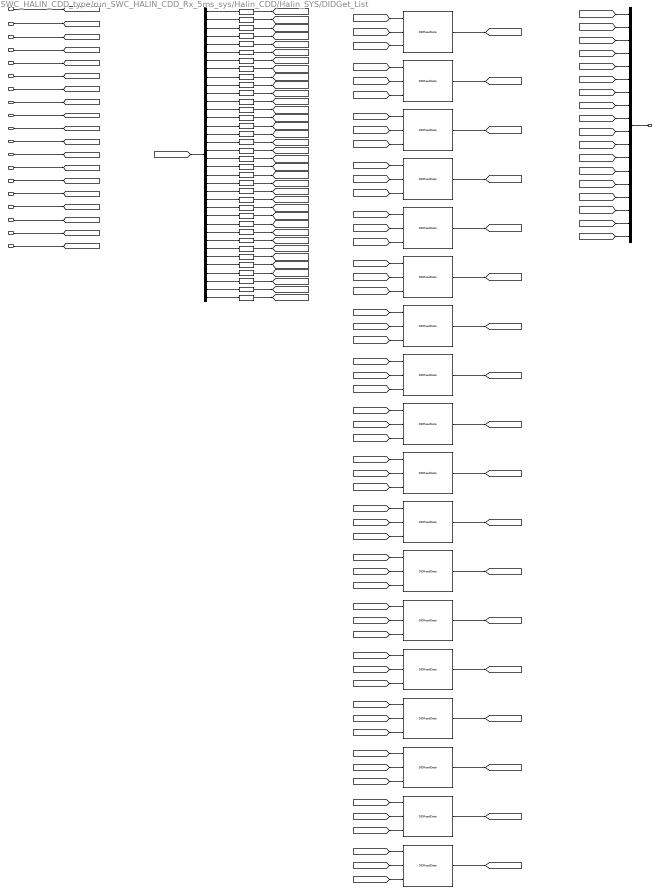
== system SWC_HALIN_CDD_type/run_SWC_HALIN_CDD_Rx_5ms_sys/Halin_CDD/Halin_SYS/DIDGet_List ==
  BHAL_DIDGetData_raw : Inport
  VHAL_DIDFlashXWDMode_raw8 : Inport  Port=2
  VHAL_DIDFlashDKCKey_raw8 : Inport  Port=3
  VHAL_DIDFlashDynoMode_raw8 : Inport  Port=4
  VHAL_DIDFlashTurnLampFRThreCurr_raw8 : Inport  Port=5
  VHAL_DIDFlashTurnLampRRThreCurr_raw8 : Inport  Port=6
  VHAL_DIDFlashTurnLampFLThreCurr_raw8 : Inport  Port=7
  VHAL_DIDFlashTurnLampRLThreCurr_raw8 : Inport  Port=8
  VHAL_DIDFlashFMHTimer_raw8 : Inport  Port=9
  VHAL_DIDFlashAutoLock_raw8 : Inport  Port=10
  VHAL_DIDFlashDRLDis_raw8 : Inport  Port=11
  VHAL_DIDFlashAutoWipHSpdEN_raw8 : Inport  Port=12
  VHAL_DIDFlashWipRLSCmdHoldFilter_raw8 : Inport  Port=13
  VHAL_DIDFlashWipRLSCmdCutFilter_raw8 : Inport  Port=14
  VHAL_DIDFlashUSSConfig_raw8 : Inport  Port=15
  VHAL_DIDFlashTireSize_raw8 : Inport  Port=16
  VHAL_DIDFlashAPSFunConfig_raw8 : Inport  Port=17
  VHAL_DIDFlashOBDReq_raw8 : Inport  Port=18
  VHAL_DIDFlashTestGroup_raw8 : Inport  Port=19
  Auto Wiper High Speed Function Enable : hcu_lib/Basic_Blocks/DIDReadData
  AutoLock : hcu_lib/Basic_Blocks/DIDReadData
  Certification Test Group : hcu_lib/Basic_Blocks/DIDReadData
  DRLDisable : hcu_lib/Basic_Blocks/DIDReadData
  Dyno mode switch : hcu_lib/Basic_Blocks/DIDReadData
  FollowMeHomeTimer : hcu_lib/Basic_Blocks/DIDReadData
  OBD requirements : hcu_lib/Basic_Blocks/DIDReadData
  TurnLampFrontLeftThresholdCurrent : hcu_lib/Basic_Blocks/DIDReadData
  TurnLampFrontRightThresholdCurrent : hcu_lib/Basic_Blocks/DIDReadData
  TurnLampRearLeftThresholdCurrent : hcu_lib/Basic_Blocks/DIDReadData
  TurnLampRearRightThresholdCurrent : hcu_lib/Basic_Blocks/DIDReadData
  UnitConverter{,1..35} (36 alike) : DataTypeConversion  OutDataTypeStr=uint8
  Wiper RLS Command Cut Filter : hcu_lib/Basic_Blocks/DIDReadData
  Wiper RLS Command Hold Filter : hcu_lib/Basic_Blocks/DIDReadData
  WriteRandomNumberDKC : hcu_lib/Basic_Blocks/DIDReadData
  XWD switch : hcu_lib/Basic_Blocks/DIDReadData
  apsFunctionConfiguration : hcu_lib/Basic_Blocks/DIDReadData
  apsUssConfiguration : hcu_lib/Basic_Blocks/DIDReadData
  apsVehicleTireSize : hcu_lib/Basic_Blocks/DIDReadData
  bus_Creator : BusCreator  Inputs=18
  bus_selector : BusSelector  OutputSignals=VHAL_DIDStaXWDMode_raw,VHAL_XWDMode_raw,VHAL_DIDStaDKCKey_raw,VHAL_DKCKey_raw,VHAL_DIDStaDynoMode_raw,VHAL_DynoMode_raw,VHAL_DIDStaTurnLampFRThreCurr_raw,VHAL_TurnLampFRThreCurr_raw,VHAL_DIDStaTurnLampRRThreCurr_raw,VHAL_TurnLampRRThreCurr_raw,VHAL_DIDStaTurnLampFLThreCurr_raw,VHAL_TurnLampFLThreCurr_raw,VHAL_DIDStaTurnLampRLThreCurr_raw,VHAL_TurnLampRLThreCurr_raw,VHAL_DIDStaFMHTimer_raw,VHAL_FMHTimer_raw,VHAL_DIDStaAutoLock_raw,VHAL_AutoLock_raw,VHAL_DIDStaDRLDis_raw,VHAL_DRLDis_raw,VHAL_DIDStaAutoWipHSpdEN_raw,VHAL_AutoWipHSpdEN_raw,VHAL_DIDStaWipRLSCmdHoldFilter_raw,VHAL_WipRLSCmdHoldFilter_raw,VHAL_DIDStaWipRLSCmdCutFilter_raw,VHAL_WipRLSCmdCutFilter_raw,VHAL_DIDStaUSSConfig_raw,VHAL_USSConfig_raw,VHAL_DIDStaTireSize_raw,VHAL_TireSize_raw,VHAL_DIDStaAPSFunConfig_raw,VHAL_APSFunConfig_raw,VHAL_DIDStaOBDReq_raw,VHAL_OBDReq_raw,VHAL_DIDStaTestGroup_raw,VHAL_TestGroup_raw
  BHAL_DIDOrigOutput_raw8 : Outport
  wires:
  BHAL_DIDGetData_raw/1 -> [BHAL_DIDGetData_raw]
  VHAL_DIDFlashXWDMode_raw8/1 -> [VHAL_DIDFlashXWDMode_raw8]
  VHAL_DIDFlashDKCKey_raw8/1 -> [VHAL_DIDFlashDKCKey_raw8]
  VHAL_DIDFlashDynoMode_raw8/1 -> [VHAL_DIDFlashDynoMode_raw8]
  VHAL_DIDFlashTurnLampFRThreCurr_raw8/1 -> [VHAL_DIDFlashTurnLampFRThreCurr_raw8]
  VHAL_DIDFlashTurnLampRRThreCurr_raw8/1 -> [VHAL_DIDFlashTurnLampRRThreCurr_raw8]
  VHAL_DIDFlashTurnLampFLThreCurr_raw8/1 -> [VHAL_DIDFlashTurnLampFLThreCurr_raw8]
  VHAL_DIDFlashTurnLampRLThreCurr_raw8/1 -> [VHAL_DIDFlashTurnLampRLThreCurr_raw8]
  VHAL_DIDFlashFMHTimer_raw8/1 -> [VHAL_DIDFlashFMHTimer_raw8]
  VHAL_DIDFlashAutoLock_raw8/1 -> [VHAL_DIDFlashAutoLock_raw8]
  VHAL_DIDFlashDRLDis_raw8/1 -> [VHAL_DIDFlashDRLDis_raw8]
  VHAL_DIDFlashAutoWipHSpdEN_raw8/1 -> [VHAL_DIDFlashAutoWipHSpdEN_raw8]
  VHAL_DIDFlashWipRLSCmdHoldFilter_raw8/1 -> [VHAL_DIDFlashWipRLSCmdHoldFilter_raw8]
  VHAL_DIDFlashWipRLSCmdCutFilter_raw8/1 -> [VHAL_DIDFlashWipRLSCmdCutFilter_raw8]
  VHAL_DIDFlashUSSConfig_raw8/1 -> [VHAL_DIDFlashUSSConfig_raw8]
  VHAL_DIDFlashTireSize_raw8/1 -> [VHAL_DIDFlashTireSize_raw8]
  VHAL_DIDFlashAPSFunConfig_raw8/1 -> [VHAL_DIDFlashAPSFunConfig_raw8]
  VHAL_DIDFlashOBDReq_raw8/1 -> [VHAL_DIDFlashOBDReq_raw8]
  VHAL_DIDFlashTestGroup_raw8/1 -> [VHAL_DIDFlashTestGroup_raw8]
  [BHAL_DIDGetData_raw] -> bus_selector/1
  bus_selector/1 -> UnitConverter/1  "<VHAL_DIDStaXWDMode_raw>"
  UnitConverter/1 -> [VHAL_DIDStaXWDMode_raw]  "VHAL_DIDStaXWDMode_raw"
  bus_selector/2 -> UnitConverter1/1  "<VHAL_XWDMode_raw>"
  UnitConverter1/1 -> [VHAL_XWDMode_raw]  "VHAL_XWDMode_raw"
  bus_selector/3 -> UnitConverter2/1  "<VHAL_DIDStaDKCKey_raw>"
  UnitConverter2/1 -> [VHAL_DIDStaDKCKey_raw]  "VHAL_DIDStaDKCKey_raw"
  bus_selector/4 -> UnitConverter3/1  "<VHAL_DKCKey_raw>"
  UnitConverter3/1 -> [VHAL_DKCKey_raw]  "VHAL_DKCKey_raw"
  bus_selector/5 -> UnitConverter4/1  "<VHAL_DIDStaDynoMode_raw>"
  UnitConverter4/1 -> [VHAL_DIDStaDynoMode_raw]  "VHAL_DIDStaDynoMode_raw"
  bus_selector/6 -> UnitConverter5/1  "<VHAL_DynoMode_raw>"
  UnitConverter5/1 -> [VHAL_DynoMode_raw]  "VHAL_DynoMode_raw"
  bus_selector/7 -> UnitConverter6/1  "<VHAL_DIDStaTurnLampFRThreCurr_raw>"
  UnitConverter6/1 -> [VHAL_DIDStaTurnLampFRThreCurr_raw]  "VHAL_DIDStaTurnLampFRThreCurr_raw"
  bus_selector/8 -> UnitConverter7/1  "<VHAL_TurnLampFRThreCurr_raw>"
  UnitConverter7/1 -> [VHAL_TurnLampFRThreCurr_raw]  "VHAL_TurnLampFRThreCurr_raw"
  bus_selector/9 -> UnitConverter8/1  "<VHAL_DIDStaTurnLampRRThreCurr_raw>"
  UnitConverter8/1 -> [VHAL_DIDStaTurnLampRRThreCurr_raw]  "VHAL_DIDStaTurnLampRRThreCurr_raw"
  bus_selector/10 -> UnitConverter9/1  "<VHAL_TurnLampRRThreCurr_raw>"
  UnitConverter9/1 -> [VHAL_TurnLampRRThreCurr_raw]  "VHAL_TurnLampRRThreCurr_raw"
  bus_selector/11 -> UnitConverter10/1  "<VHAL_DIDStaTurnLampFLThreCurr_raw>"
  UnitConverter10/1 -> [VHAL_DIDStaTurnLampFLThreCurr_raw]  "VHAL_DIDStaTurnLampFLThreCurr_raw"
  bus_selector/12 -> UnitConverter11/1  "<VHAL_TurnLampFLThreCurr_raw>"
  UnitConverter11/1 -> [VHAL_TurnLampFLThreCurr_raw]  "VHAL_TurnLampFLThreCurr_raw"
  bus_selector/13 -> UnitConverter12/1  "<VHAL_DIDStaTurnLampRLThreCurr_raw>"
  UnitConverter12/1 -> [VHAL_DIDStaTurnLampRLThreCurr_raw]  "VHAL_DIDStaTurnLampRLThreCurr_raw"
  bus_selector/14 -> UnitConverter13/1  "<VHAL_TurnLampRLThreCurr_raw>"
  UnitConverter13/1 -> [VHAL_TurnLampRLThreCurr_raw]  "VHAL_TurnLampRLThreCurr_raw"
  bus_selector/15 -> UnitConverter14/1  "<VHAL_DIDStaFMHTimer_raw>"
  UnitConverter14/1 -> [VHAL_DIDStaFMHTimer_raw]  "VHAL_DIDStaFMHTimer_raw"
  bus_selector/16 -> UnitConverter15/1  "<VHAL_FMHTimer_raw>"
  UnitConverter15/1 -> [VHAL_FMHTimer_raw]  "VHAL_FMHTimer_raw"
  bus_selector/17 -> UnitConverter16/1  "<VHAL_DIDStaAutoLock_raw>"
  UnitConverter16/1 -> [VHAL_DIDStaAutoLock_raw]  "VHAL_DIDStaAutoLock_raw"
  bus_selector/18 -> UnitConverter17/1  "<VHAL_AutoLock_raw>"
  UnitConverter17/1 -> [VHAL_AutoLock_raw]  "VHAL_AutoLock_raw"
  bus_selector/19 -> UnitConverter18/1  "<VHAL_DIDStaDRLDis_raw>"
  UnitConverter18/1 -> [VHAL_DIDStaDRLDis_raw]  "VHAL_DIDStaDRLDis_raw"
  bus_selector/20 -> UnitConverter19/1  "<VHAL_DRLDis_raw>"
  UnitConverter19/1 -> [VHAL_DRLDis_raw]  "VHAL_DRLDis_raw"
  bus_selector/21 -> UnitConverter20/1  "<VHAL_DIDStaAutoWipHSpdEN_raw>"
  UnitConverter20/1 -> [VHAL_DIDStaAutoWipHSpdEN_raw]  "VHAL_DIDStaAutoWipHSpdEN_raw"
  bus_selector/22 -> UnitConverter21/1  "<VHAL_AutoWipHSpdEN_raw>"
  UnitConverter21/1 -> [VHAL_AutoWipHSpdEN_raw]  "VHAL_AutoWipHSpdEN_raw"
  bus_selector/23 -> UnitConverter22/1  "<VHAL_DIDStaWipRLSCmdHoldFilter_raw>"
  UnitConverter22/1 -> [VHAL_DIDStaWipRLSCmdHoldFilter_raw]  "VHAL_DIDStaWipRLSCmdHoldFilter_raw"
  bus_selector/24 -> UnitConverter23/1  "<VHAL_WipRLSCmdHoldFilter_raw>"
  UnitConverter23/1 -> [VHAL_WipRLSCmdHoldFilter_raw]  "VHAL_WipRLSCmdHoldFilter_raw"
  bus_selector/25 -> UnitConverter24/1  "<VHAL_DIDStaWipRLSCmdCutFilter_raw>"
  UnitConverter24/1 -> [VHAL_DIDStaWipRLSCmdCutFilter_raw]  "VHAL_DIDStaWipRLSCmdCutFilter_raw"
  bus_selector/26 -> UnitConverter25/1  "<VHAL_WipRLSCmdCutFilter_raw>"
  UnitConverter25/1 -> [VHAL_WipRLSCmdCutFilter_raw]  "VHAL_WipRLSCmdCutFilter_raw"
  bus_selector/27 -> UnitConverter26/1  "<VHAL_DIDStaUSSConfig_raw>"
  UnitConverter26/1 -> [VHAL_DIDStaUSSConfig_raw]  "VHAL_DIDStaUSSConfig_raw"
  bus_selector/28 -> UnitConverter27/1  "<VHAL_USSConfig_raw>"
  UnitConverter27/1 -> [VHAL_USSConfig_raw]  "VHAL_USSConfig_raw"
  bus_selector/29 -> UnitConverter28/1  "<VHAL_DIDStaTireSize_raw>"
  UnitConverter28/1 -> [VHAL_DIDStaTireSize_raw]  "VHAL_DIDStaTireSize_raw"
  bus_selector/30 -> UnitConverter29/1  "<VHAL_TireSize_raw>"
  UnitConverter29/1 -> [VHAL_TireSize_raw]  "VHAL_TireSize_raw"
  bus_selector/31 -> UnitConverter30/1  "<VHAL_DIDStaAPSFunConfig_raw>"
  UnitConverter30/1 -> [VHAL_DIDStaAPSFunConfig_raw]  "VHAL_DIDStaAPSFunConfig_raw"
  bus_selector/32 -> UnitConverter31/1  "<VHAL_APSFunConfig_raw>"
  UnitConverter31/1 -> [VHAL_APSFunConfig_raw]  "VHAL_APSFunConfig_raw"
  bus_selector/33 -> UnitConverter32/1  "<VHAL_DIDStaOBDReq_raw>"
  UnitConverter32/1 -> [VHAL_DIDStaOBDReq_raw]  "VHAL_DIDStaOBDReq_raw"
  bus_selector/34 -> UnitConverter33/1  "<VHAL_OBDReq_raw>"
  UnitConverter33/1 -> [VHAL_OBDReq_raw]  "VHAL_OBDReq_raw"
  bus_selector/35 -> UnitConverter34/1  "<VHAL_DIDStaTestGroup_raw>"
  UnitConverter34/1 -> [VHAL_DIDStaTestGroup_raw]  "VHAL_DIDStaTestGroup_raw"
  bus_selector/36 -> UnitConverter35/1  "<VHAL_TestGroup_raw>"
  UnitConverter35/1 -> [VHAL_TestGroup_raw]  "VHAL_TestGroup_raw"
  [VHAL_XWDMode_raw] -> XWD switch/1
  [VHAL_DIDStaXWDMode_raw] -> XWD switch/2
  [VHAL_DIDFlashXWDMode_raw8] -> XWD switch/3
  XWD switch/1 -> [VHAL_DIDGetXWDMode_raw8]
  [VHAL_DKCKey_raw] -> WriteRandomNumberDKC/1
  [VHAL_DIDStaDKCKey_raw] -> WriteRandomNumberDKC/2
  [VHAL_DIDFlashDKCKey_raw8] -> WriteRandomNumberDKC/3
  WriteRandomNumberDKC/1 -> [VHAL_DIDGetDKCKey_raw8]
  [VHAL_DynoMode_raw] -> Dyno mode switch/1
  [VHAL_DIDStaDynoMode_raw] -> Dyno mode switch/2
  [VHAL_DIDFlashDynoMode_raw8] -> Dyno mode switch/3
  Dyno mode switch/1 -> [VHAL_DIDGetDynoMode_raw8]
  [VHAL_TurnLampFRThreCurr_raw] -> TurnLampFrontRightThresholdCurrent/1
  [VHAL_DIDStaTurnLampFRThreCurr_raw] -> TurnLampFrontRightThresholdCurrent/2
  [VHAL_DIDFlashTurnLampFRThreCurr_raw8] -> TurnLampFrontRightThresholdCurrent/3
  TurnLampFrontRightThresholdCurrent/1 -> [VHAL_DIDGetTurnLampFRThreCurr_raw8]
  [VHAL_TurnLampRRThreCurr_raw] -> TurnLampRearRightThresholdCurrent/1
  [VHAL_DIDStaTurnLampRRThreCurr_raw] -> TurnLampRearRightThresholdCurrent/2
  [VHAL_DIDFlashTurnLampRRThreCurr_raw8] -> TurnLampRearRightThresholdCurrent/3
  TurnLampRearRightThresholdCurrent/1 -> [VHAL_DIDGetTurnLampRRThreCurr_raw8]
  [VHAL_TurnLampFLThreCurr_raw] -> TurnLampFrontLeftThresholdCurrent/1
  [VHAL_DIDStaTurnLampFLThreCurr_raw] -> TurnLampFrontLeftThresholdCurrent/2
  [VHAL_DIDFlashTurnLampFLThreCurr_raw8] -> TurnLampFrontLeftThresholdCurrent/3
  TurnLampFrontLeftThresholdCurrent/1 -> [VHAL_DIDGetTurnLampFLThreCurr_raw8]
  [VHAL_TurnLampRLThreCurr_raw] -> TurnLampRearLeftThresholdCurrent/1
  [VHAL_DIDStaTurnLampRLThreCurr_raw] -> TurnLampRearLeftThresholdCurrent/2
  [VHAL_DIDFlashTurnLampRLThreCurr_raw8] -> TurnLampRearLeftThresholdCurrent/3
  TurnLampRearLeftThresholdCurrent/1 -> [VHAL_DIDGetTurnLampRLThreCurr_raw8]
  [VHAL_FMHTimer_raw] -> FollowMeHomeTimer/1
  [VHAL_DIDStaFMHTimer_raw] -> FollowMeHomeTimer/2
  [VHAL_DIDFlashFMHTimer_raw8] -> FollowMeHomeTimer/3
  FollowMeHomeTimer/1 -> [VHAL_DIDGetFMHTimer_raw8]
  [VHAL_AutoLock_raw] -> AutoLock/1
  [VHAL_DIDStaAutoLock_raw] -> AutoLock/2
  [VHAL_DIDFlashAutoLock_raw8] -> AutoLock/3
  AutoLock/1 -> [VHAL_DIDGetAutoLock_raw8]
  [VHAL_DRLDis_raw] -> DRLDisable/1
  [VHAL_DIDStaDRLDis_raw] -> DRLDisable/2
  [VHAL_DIDFlashDRLDis_raw8] -> DRLDisable/3
  DRLDisable/1 -> [VHAL_DIDGetDRLDis_raw8]
  [VHAL_AutoWipHSpdEN_raw] -> Auto Wiper High Speed Function Enable/1
  [VHAL_DIDStaAutoWipHSpdEN_raw] -> Auto Wiper High Speed Function Enable/2
  [VHAL_DIDFlashAutoWipHSpdEN_raw8] -> Auto Wiper High Speed Function Enable/3
  Auto Wiper High Speed Function Enable/1 -> [VHAL_DIDGetAutoWipHSpdEN_raw8]
  [VHAL_WipRLSCmdHoldFilter_raw] -> Wiper RLS Command Hold Filter/1
  [VHAL_DIDStaWipRLSCmdHoldFilter_raw] -> Wiper RLS Command Hold Filter/2
  [VHAL_DIDFlashWipRLSCmdHoldFilter_raw8] -> Wiper RLS Command Hold Filter/3
  Wiper RLS Command Hold Filter/1 -> [VHAL_DIDGetWipRLSCmdHoldFilter_raw8]
  [VHAL_WipRLSCmdCutFilter_raw] -> Wiper RLS Command Cut Filter/1
  [VHAL_DIDStaWipRLSCmdCutFilter_raw] -> Wiper RLS Command Cut Filter/2
  [VHAL_DIDFlashWipRLSCmdCutFilter_raw8] -> Wiper RLS Command Cut Filter/3
  Wiper RLS Command Cut Filter/1 -> [VHAL_DIDGetWipRLSCmdCutFilter_raw8]
  [VHAL_USSConfig_raw] -> apsUssConfiguration/1
  [VHAL_DIDStaUSSConfig_raw] -> apsUssConfiguration/2
  [VHAL_DIDFlashUSSConfig_raw8] -> apsUssConfiguration/3
  apsUssConfiguration/1 -> [VHAL_DIDGetUSSConfig_raw8]
  [VHAL_TireSize_raw] -> apsVehicleTireSize/1
  [VHAL_DIDStaTireSize_raw] -> apsVehicleTireSize/2
  [VHAL_DIDFlashTireSize_raw8] -> apsVehicleTireSize/3
  apsVehicleTireSize/1 -> [VHAL_DIDGetTireSize_raw8]
  [VHAL_APSFunConfig_raw] -> apsFunctionConfiguration/1
  [VHAL_DIDStaAPSFunConfig_raw] -> apsFunctionConfiguration/2
  [VHAL_DIDFlashAPSFunConfig_raw8] -> apsFunctionConfiguration/3
  apsFunctionConfiguration/1 -> [VHAL_DIDGetAPSFunConfig_raw8]
  [VHAL_OBDReq_raw] -> OBD requirements/1
  [VHAL_DIDStaOBDReq_raw] -> OBD requirements/2
  [VHAL_DIDFlashOBDReq_raw8] -> OBD requirements/3
  OBD requirements/1 -> [VHAL_DIDGetOBDReq_raw8]
  [VHAL_TestGroup_raw] -> Certification Test Group/1
  [VHAL_DIDStaTestGroup_raw] -> Certification Test Group/2
  [VHAL_DIDFlashTestGroup_raw8] -> Certification Test Group/3
  Certification Test Group/1 -> [VHAL_DIDGetTestGroup_raw8]
  [VHAL_DIDGetXWDMode_raw8] -> bus_Creator/1  "VHAL_DIDGetXWDMode_raw8"
  [VHAL_DIDGetDKCKey_raw8] -> bus_Creator/2  "VHAL_DIDGetDKCKey_raw8"
  [VHAL_DIDGetDynoMode_raw8] -> bus_Creator/3  "VHAL_DIDGetDynoMode_raw8"
  [VHAL_DIDGetTurnLampFRThreCurr_raw8] -> bus_Creator/4  "VHAL_DIDGetTurnLampFRThreCurr_raw8"
  [VHAL_DIDGetTurnLampRRThreCurr_raw8] -> bus_Creator/5  "VHAL_DIDGetTurnLampRRThreCurr_raw8"
  [VHAL_DIDGetTurnLampFLThreCurr_raw8] -> bus_Creator/6  "VHAL_DIDGetTurnLampFLThreCurr_raw8"
  [VHAL_DIDGetTurnLampRLThreCurr_raw8] -> bus_Creator/7  "VHAL_DIDGetTurnLampRLThreCurr_raw8"
  [VHAL_DIDGetFMHTimer_raw8] -> bus_Creator/8  "VHAL_DIDGetFMHTimer_raw8"
  [VHAL_DIDGetAutoLock_raw8] -> bus_Creator/9  "VHAL_DIDGetAutoLock_raw8"
  [VHAL_DIDGetDRLDis_raw8] -> bus_Creator/10  "VHAL_DIDGetDRLDis_raw8"
  [VHAL_DIDGetAutoWipHSpdEN_raw8] -> bus_Creator/11  "VHAL_DIDGetAutoWipHSpdEN_raw8"
  [VHAL_DIDGetWipRLSCmdHoldFilter_raw8] -> bus_Creator/12  "VHAL_DIDGetWipRLSCmdHoldFilter_raw8"
  [VHAL_DIDGetWipRLSCmdCutFilter_raw8] -> bus_Creator/13  "VHAL_DIDGetWipRLSCmdCutFilter_raw8"
  [VHAL_DIDGetUSSConfig_raw8] -> bus_Creator/14  "VHAL_DIDGetUSSConfig_raw8"
  [VHAL_DIDGetTireSize_raw8] -> bus_Creator/15  "VHAL_DIDGetTireSize_raw8"
  [VHAL_DIDGetAPSFunConfig_raw8] -> bus_Creator/16  "VHAL_DIDGetAPSFunConfig_raw8"
  [VHAL_DIDGetOBDReq_raw8] -> bus_Creator/17  "VHAL_DIDGetOBDReq_raw8"
  [VHAL_DIDGetTestGroup_raw8] -> bus_Creator/18  "VHAL_DIDGetTestGroup_raw8"
  bus_Creator/1 -> BHAL_DIDOrigOutput_raw8/1

== system SWC_HALIN_CDD_type/run_SWC_HALIN_CDD_Rx_5ms_sys/Halin_CDD/Halin_SYS/FlashACForceOFF_Verify ==
  In1 : Inport
  Compare To Constant : simulink/Logic and Bit Operations/Compare To Constant  relop=>  const=1  OutDataTypeStr=boolean
  Compare To Constant1 : simulink/Logic and Bit Operations/Compare To Constant  relop=<  const=0  OutDataTypeStr=boolean
  Constant : Constant  Value=ZERO_INT
  Logical Operator : Logic  Operator=OR  AllPortsSameDT=off  OutDataTypeStr=boolean
  Switch : Switch  Criteria=u2 > Threshold
  Out1 : Outport
  wires:
  In1/1 -> Switch/3, Compare To Constant1/1, Compare To Constant/1
  Constant/1 -> Switch/1
  Switch/1 -> Out1/1
  Logical Operator/1 -> Switch/2
  Compare To Constant/1 -> Logical Operator/1
  Compare To Constant1/1 -> Logical Operator/2

== system SWC_HALIN_CDD_type/run_SWC_HALIN_CDD_Rx_5ms_sys/Halin_CDD/Halin_SYS/FlashAPMDoorControlSta ==
  In1 : Inport
  Compare To Constant : simulink/Logic and Bit Operations/Compare To Constant  relop=>  const=1  OutDataTypeStr=boolean
  Compare To Constant1 : simulink/Logic and Bit Operations/Compare To Constant  relop=<  const=0  OutDataTypeStr=boolean
  Constant : Constant  Value=ONE_INT
  Logical Operator : Logic  Operator=OR  AllPortsSameDT=off  OutDataTypeStr=boolean
  Switch : Switch  Criteria=u2 > Threshold
  Out1 : Outport
  wires:
  In1/1 -> Switch/3, Compare To Constant1/1, Compare To Constant/1
  Constant/1 -> Switch/1
  Switch/1 -> Out1/1
  Logical Operator/1 -> Switch/2
  Compare To Constant/1 -> Logical Operator/1
  Compare To Constant1/1 -> Logical Operator/2

== system SWC_HALIN_CDD_type/run_SWC_HALIN_CDD_Rx_5ms_sys/Halin_CDD/Halin_SYS/FlashAirIntenZone1M_Verify ==
  In1 : Inport
  Compare To Constant : simulink/Logic and Bit Operations/Compare To Constant  relop=>  const=15  OutDataTypeStr=boolean
  Compare To Constant1 : simulink/Logic and Bit Operations/Compare To Constant  relop=<  const=1  OutDataTypeStr=boolean
  Constant : Constant  Value=ONE_INT
  Logical Operator : Logic  Operator=OR  AllPortsSameDT=off  OutDataTypeStr=boolean
  Switch : Switch  Criteria=u2 > Threshold
  Out1 : Outport
  wires:
  Compare To Constant1/1 -> Logical Operator/2
  Compare To Constant/1 -> Logical Operator/1
  Logical Operator/1 -> Switch/2
  Switch/1 -> Out1/1
  Constant/1 -> Switch/1
  In1/1 -> Compare To Constant/1, Compare To Constant1/1, Switch/3

== system SWC_HALIN_CDD_type/run_SWC_HALIN_CDD_Rx_5ms_sys/Halin_CDD/Halin_SYS/FlashCountAlarm_Verify ==
  In1 : Inport
  Compare To Constant : simulink/Logic and Bit Operations/Compare To Constant  relop=>  const=15  OutDataTypeStr=boolean
  Compare To Constant1 : simulink/Logic and Bit Operations/Compare To Constant  relop=<  const=0  OutDataTypeStr=boolean
  Constant : Constant  Value=ZERO_INT
  Logical Operator : Logic  Operator=OR  AllPortsSameDT=off  OutDataTypeStr=boolean
  Switch : Switch  Criteria=u2 > Threshold
  Out1 : Outport
  wires:
  In1/1 -> Switch/3, Compare To Constant1/1, Compare To Constant/1
  Constant/1 -> Switch/1
  Switch/1 -> Out1/1
  Logical Operator/1 -> Switch/2
  Compare To Constant/1 -> Logical Operator/1
  Compare To Constant1/1 -> Logical Operator/2

== system SWC_HALIN_CDD_type/run_SWC_HALIN_CDD_Rx_5ms_sys/Halin_CDD/Halin_SYS/FlashFuelDoorPos_Verify ==
  In1 : Inport
  Compare To Constant : simulink/Logic and Bit Operations/Compare To Constant  relop=>  const=1  OutDataTypeStr=boolean
  Compare To Constant1 : simulink/Logic and Bit Operations/Compare To Constant  relop=<  const=0  OutDataTypeStr=boolean
  Constant : Constant  Value=ZERO_INT
  Logical Operator : Logic  Operator=OR  AllPortsSameDT=off  OutDataTypeStr=boolean
  Switch : Switch  Criteria=u2 > Threshold
  Out1 : Outport
  wires:
  Compare To Constant1/1 -> Logical Operator/2
  Compare To Constant/1 -> Logical Operator/1
  Logical Operator/1 -> Switch/2
  Switch/1 -> Out1/1
  Constant/1 -> Switch/1
  In1/1 -> Compare To Constant/1, Compare To Constant1/1, Switch/3

== system SWC_HALIN_CDD_type/run_SWC_HALIN_CDD_Rx_5ms_sys/Halin_CDD/Halin_SYS/FlashIVIPTGUSStaSW_Verify ==
  In1 : Inport
  Compare To Constant : simulink/Logic and Bit Operations/Compare To Constant  relop=>  const=1  OutDataTypeStr=boolean
  Compare To Constant1 : simulink/Logic and Bit Operations/Compare To Constant  relop=<  const=0  OutDataTypeStr=boolean
  Constant : Constant  Value=ZERO_INT
  Logical Operator : Logic  Operator=OR  AllPortsSameDT=off  OutDataTypeStr=boolean
  Switch : Switch  Criteria=u2 > Threshold
  Out1 : Outport
  wires:
  In1/1 -> Switch/3, Compare To Constant1/1, Compare To Constant/1
  Constant/1 -> Switch/1
  Switch/1 -> Out1/1
  Logical Operator/1 -> Switch/2
  Compare To Constant/1 -> Logical Operator/1
  Compare To Constant1/1 -> Logical Operator/2

== system SWC_HALIN_CDD_type/run_SWC_HALIN_CDD_Rx_5ms_sys/Halin_CDD/Halin_SYS/FlashMFRDNBrightReq_Verify ==
  In1 : Inport
  Compare To Constant : simulink/Logic and Bit Operations/Compare To Constant  relop=>  const=127  OutDataTypeStr=boolean
  Compare To Constant1 : simulink/Logic and Bit Operations/Compare To Constant  relop=<  const=0  OutDataTypeStr=boolean
  Constant : Constant  Value=ZERO_INT
  Logical Operator : Logic  Operator=OR  AllPortsSameDT=off  OutDataTypeStr=boolean
  Switch : Switch  Criteria=u2 > Threshold
  Out1 : Outport
  wires:
  Compare To Constant1/1 -> Logical Operator/2
  Compare To Constant/1 -> Logical Operator/1
  Logical Operator/1 -> Switch/2
  Switch/1 -> Out1/1
  Constant/1 -> Switch/1
  In1/1 -> Compare To Constant/1, Compare To Constant1/1, Switch/3
